simulink model "PowerWindowControl_V6"  (R2021a)
settings: Solver=VariableStepAuto  StartTime=0.0  StopTime=40  RelTol=1e-3
model workspace (MATLAB code in the model file):
  | testing=1;
undefined symbols (not defined in the file): sigbuilder_block
settings Model: VariantConfigurationObject=input_variant  EnablePacing=on  PacingRate=0.630000  Creator=achu  LastModifiedBy=achu

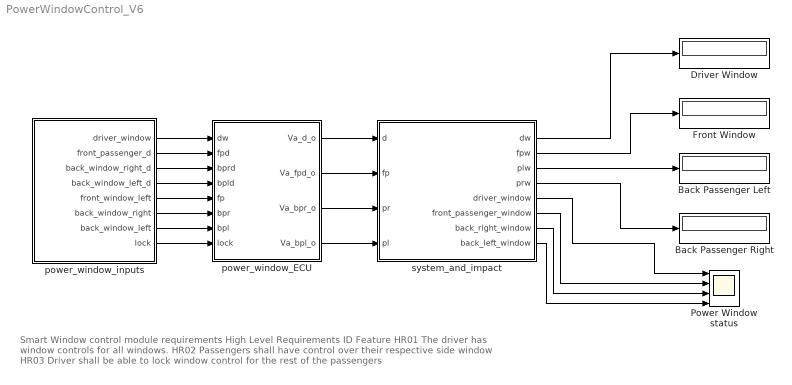
== system PowerWindowControl_V6 ==
  note: Smart Window control module requirements
      |
      | High Level Requirements
      |
      | ID
      | Feature
      |
      | HR01
      | The driver has window controls for all windows.
      |
      | HR02
      | Passengers shall have control over their respective side window
      |
      | HR03
      | Driver shall be able to lock window control for the rest of the passengers
  Back Passenger Left : Display
  Back Passenger Right : Display
  Driver Window : Display
  Front Window : Display
  Power Window status : Scope  NumInputPorts=4
  power_window_ECU : Subsystem
  power_window_inputs : Subsystem
  system_and_impact : Subsystem
  wires:
  system_and_impact/1(dw) -> Driver Window/1
  system_and_impact/4(prw) -> Back Passenger Right/1
  system_and_impact/2(fpw) -> Front Window/1
  system_and_impact/3(plw) -> Back Passenger Left/1
  system_and_impact/6(front_passenger_window) -> Power Window status/2
  system_and_impact/5(driver_window) -> Power Window status/1
  system_and_impact/7(back_right_window) -> Power Window status/3
  system_and_impact/8(back_left_window) -> Power Window status/4
  power_window_ECU/1(Va_d_o) -> system_and_impact/1(d)
  power_window_ECU/2(Va_fpd_o) -> system_and_impact/2(fp)
  power_window_ECU/3(Va_bpr_o) -> system_and_impact/3(pr)
  power_window_ECU/4(Va_bpl_o) -> system_and_impact/4(pl)
  power_window_inputs/1(driver_window) -> power_window_ECU/1(dw)
  power_window_inputs/2(front_passenger_d) -> power_window_ECU/2(fpd)
  power_window_inputs/3(back_window_right_d) -> power_window_ECU/3(bprd)
  power_window_inputs/4(back_window_left_d) -> power_window_ECU/4(bpld)
  power_window_inputs/5(front_window_left) -> power_window_ECU/5(fp)
  power_window_inputs/6(back_window_right) -> power_window_ECU/6(bpr)
  power_window_inputs/7(back_window_left) -> power_window_ECU/7(bpl)
  power_window_inputs/8(lock) -> power_window_ECU/8(lock)

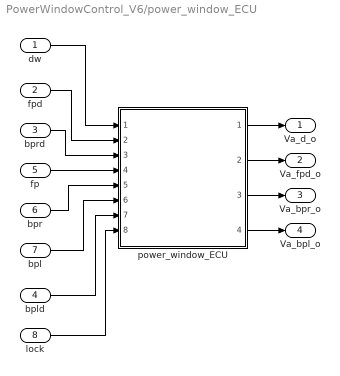
== system PowerWindowControl_V6/power_window_ECU ==
  dw : Inport
  fpd : Inport  Port=2
  bprd : Inport  Port=3
  bpld : Inport  Port=4
  fp : Inport  Port=5
  bpr : Inport  Port=6
  bpl : Inport  Port=7
  lock : Inport  Port=8
  power_window_ECU : Subsystem  ReferencedSubsystem=power_windows_ECU
  Va_d_o : Outport
  Va_fpd_o : Outport  Port=2
  Va_bpr_o : Outport  Port=3
  Va_bpl_o : Outport  Port=4
  wires:
  fp/1 -> power_window_ECU/4
  power_window_ECU/4 -> Va_bpl_o/1
  bprd/1 -> power_window_ECU/3
  dw/1 -> power_window_ECU/1
  bpr/1 -> power_window_ECU/5
  fpd/1 -> power_window_ECU/2
  power_window_ECU/2 -> Va_fpd_o/1
  lock/1 -> power_window_ECU/8
  bpl/1 -> power_window_ECU/6
  bpld/1 -> power_window_ECU/7
  power_window_ECU/3 -> Va_bpr_o/1
  power_window_ECU/1 -> Va_d_o/1

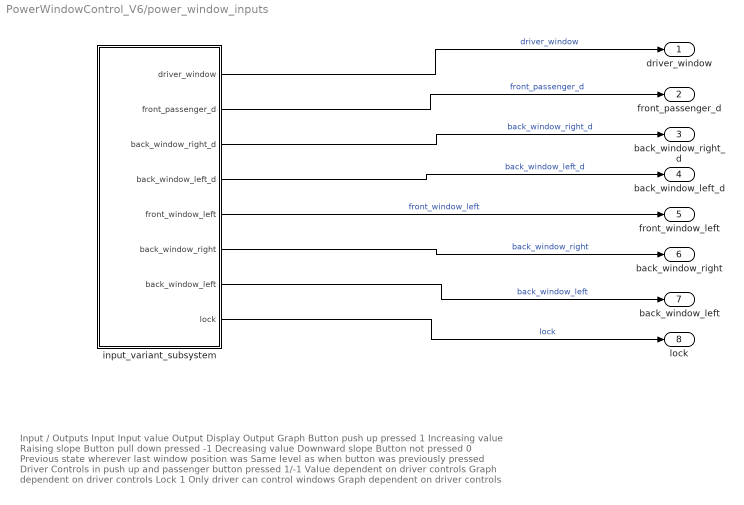
== system PowerWindowControl_V6/power_window_inputs ==
  note: Input / Outputs
      |
      | Input
      | Input value
      | Output Display
      | Output Graph
      |
      | Button push up pressed
      | 1
      | Increasing value
      | Raising slope
      |
      | Button pull down pressed
      | -1
      | Decreasing value
      | Downward slope
      |
      | Button not pressed
      | 0
      | Previous state wherever last window position was
      | Same level as when button was previously pressed
      |
      | Driver Controls in push up and passenger button pressed
      | 1/-1
      | Value dependent on driver controls
      | Graph dependent on driver controls
      |
      | Lock
      | 1
      | Only driver can control windows
      | Graph dependent on driver controls
  input_variant_subsystem : Subsystem  Variant=on
  driver_window : Outport
  front_passenger_d : Outport  Port=2
  back_window_right_d : Outport  Port=3
  back_window_left_d : Outport  Port=4
  front_window_left : Outport  Port=5
  back_window_right : Outport  Port=6
  back_window_left : Outport  Port=7
  lock : Outport  Port=8
  wires:
  input_variant_subsystem/4(back_window_left_d) -> back_window_left_d/1  "back_window_left_d"
  input_variant_subsystem/6(back_window_right) -> back_window_right/1  "back_window_right"
  input_variant_subsystem/7(back_window_left) -> back_window_left/1  "back_window_left"
  input_variant_subsystem/1(driver_window) -> driver_window/1  "driver_window"
  input_variant_subsystem/5(front_window_left) -> front_window_left/1  "front_window_left"
  input_variant_subsystem/3(back_window_right_d) -> back_window_right_d/1  "back_window_right_d"
  input_variant_subsystem/8(lock) -> lock/1  "lock"
  input_variant_subsystem/2(front_passenger_d) -> front_passenger_d/1  "front_passenger_d"

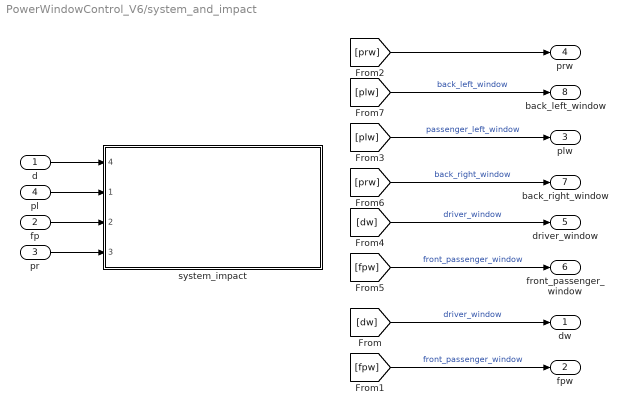
== system PowerWindowControl_V6/system_and_impact ==
  d : Inport
  fp : Inport  Port=2
  pr : Inport  Port=3
  pl : Inport  Port=4
  system_impact : Subsystem  ReferencedSubsystem=power_window_system_impact
      settings: PortSchema="{\"entries\":[{\"content\":{\"sides\":[{\"content\":{\"connectorIds\":[\"In4\",\"In1\",\"In2\",\"In3\"]},\"type\":\"ConnectorPlacement.EquallySpacedRectSide\",\"uuid\":\"b569c369-6bf1-43ff-8879-a618619a733c\"},{\"content\":{\"connectorIds\":[],\"side\":\"RIGHT\"},\"type\":\"ConnectorPlacement.EquallySpacedRectSide\",\"uuid\":\"d2d8ce62-aa5e-467c-813a-b2eb407d7f29\"},{\"content\":{\"connectorIds\":[],\"side\":\"TOP\"},\"type\":\"ConnectorPlacement.EquallySpacedRectSide\",\"uuid\":\"ba3f0d8f-c0c9-48ab-af13-329858e1637f\"}]},\"type\":\"ConnectorPlacement.EquallySpacedConnector\",\"uuid\":\"856bf121-72aa-430a-8fbb-3ccc8c554556\"}],\"packageUris\":[\"http://schema.mathworks.com/mf0/Connector/R2020b\"],\"version\":\"1.0\"}"
  dw : Outport
  fpw : Outport  Port=2
  plw : Outport  Port=3
  prw : Outport  Port=4
  driver_window : Outport  Port=5
  front_passenger_window : Outport  Port=6
  back_right_window : Outport  Port=7
  back_left_window : Outport  Port=8
  wires:
  [fpw] -> fpw/1  "front_passenger_window"
  [prw] -> back_right_window/1  "back_right_window"
  [plw] -> plw/1  "passenger_left_window"
  [dw] -> dw/1  "driver_window"
  [prw] -> prw/1
  [dw] -> driver_window/1  "driver_window"
  [plw] -> back_left_window/1  "back_left_window"
  [fpw] -> front_passenger_window/1  "front_passenger_window"
  pr/1 -> system_impact/3
  fp/1 -> system_impact/2
  pl/1 -> system_impact/1
  d/1 -> system_impact/4

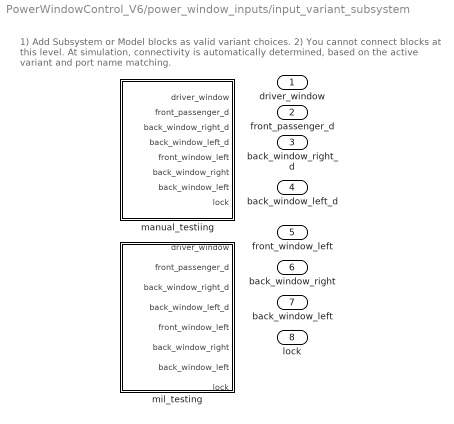
== system PowerWindowControl_V6/power_window_inputs/input_variant_subsystem ==
  note: 1) Add Subsystem or Model blocks as valid variant choices.
      | 2) You cannot connect blocks at this level. At simulation, connectivity is automatically
      | determined, based on the active variant and port name matching.
  manual_testiing : Subsystem  VariantControl=Choice
  mil_testing : Subsystem  VariantControl=Choice_1
  driver_window : Outport
  front_passenger_d : Outport  Port=2
  back_window_right_d : Outport  Port=3
  back_window_left_d : Outport  Port=4
  front_window_left : Outport  Port=5
  back_window_right : Outport  Port=6
  back_window_left : Outport  Port=7
  lock : Outport  Port=8

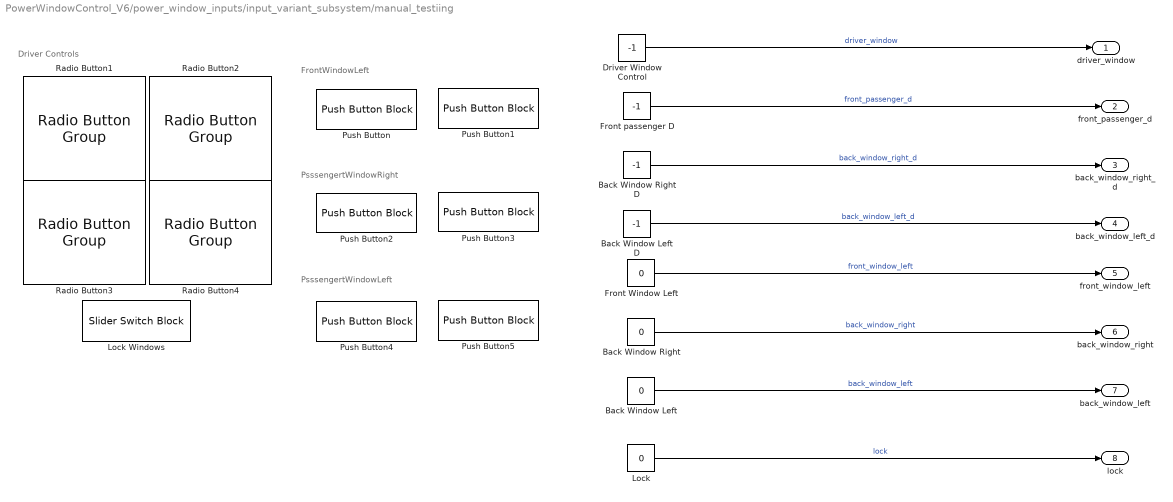
== system PowerWindowControl_V6/power_window_inputs/input_variant_subsystem/manual_testiing ==
  note: PsssengertWindowLeft
  note: PsssengertWindowRight
  note: Driver Controls
  note: FrontWindowLeft
  Back Window Left : Constant  Value=0
  Back Window Left D : Constant  Value=-1
  Back Window Right : Constant  Value=0
  Back Window Right D : Constant  Value=-1
  Driver Window Control : Constant  Value=-1
  Front Window Left : Constant  Value=0
  Front passenger D : Constant  Value=-1
  Lock : Constant  Value=0
  Lock Windows : SliderSwitchBlock
      settings: Values={{'Unlock', 'Lock'}, [0 1]}
  Push Button : PushButtonBlock  ButtonText=Push up window
  Push Button1 : PushButtonBlock  ButtonText=Pull down window  OnValue=-1
  Push Button2 : PushButtonBlock  ButtonText=Push up window
  Push Button3 : PushButtonBlock  ButtonText=Pull down window  OnValue=-1
  Push Button4 : PushButtonBlock  ButtonText=Push up window
  Push Button5 : PushButtonBlock  ButtonText=Pull down window  OnValue=-1
  Radio Button1 : RadioButtonGroup  LabelPosition=Hide  SelectedLabel=Close  ButtonGroupName=Driver Window Controls
      settings: Values={{'Open', 'Stop', 'Close'}, [1 0 -1]}
  Radio Button2 : RadioButtonGroup  LabelPosition=Hide  SelectedLabel=Close  ButtonGroupName=Front Passenger
      settings: Values={{'Open', 'Stop', 'Close'}, [1 0 -1]}
  Radio Button3 : RadioButtonGroup  LabelPosition=Hide  SelectedLabel=Close  ButtonGroupName=Back Window Right
      settings: Values={{'Open', 'Stop', 'Close'}, [1 0 -1]}
  Radio Button4 : RadioButtonGroup  LabelPosition=Hide  SelectedLabel=Close  ButtonGroupName=Back Window Left
      settings: Values={{'Open', 'Stop', 'Close'}, [1 0 -1]}
  driver_window : Outport
  front_passenger_d : Outport  Port=2
  back_window_right_d : Outport  Port=3
  back_window_left_d : Outport  Port=4
  front_window_left : Outport  Port=5
  back_window_right : Outport  Port=6
  back_window_left : Outport  Port=7
  lock : Outport  Port=8
  wires:
  Front passenger D/1 -> front_passenger_d/1  "front_passenger_d"
  Lock/1 -> lock/1  "lock"
  Front Window Left/1 -> front_window_left/1  "front_window_left"
  Driver Window Control/1 -> driver_window/1  "driver_window"
  Back Window Right D/1 -> back_window_right_d/1  "back_window_right_d"
  Back Window Left/1 -> back_window_left/1  "back_window_left"
  Back Window Right/1 -> back_window_right/1  "back_window_right"
  Back Window Left D/1 -> back_window_left_d/1  "back_window_left_d"

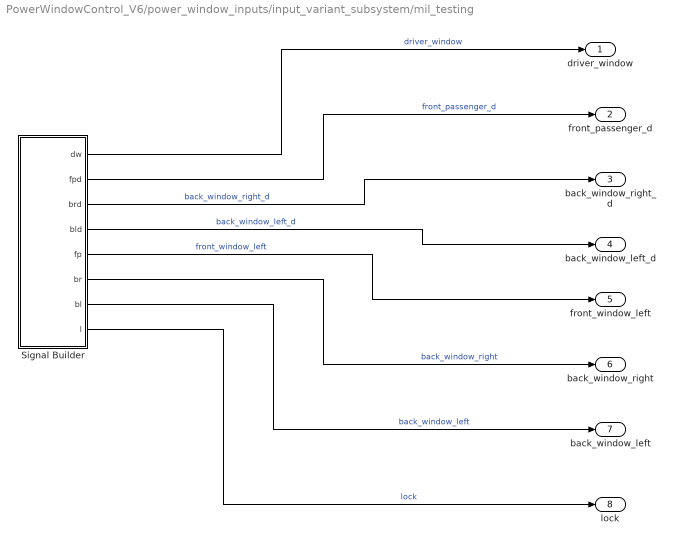
== system PowerWindowControl_V6/power_window_inputs/input_variant_subsystem/mil_testing ==
  Signal Builder : Subsystem  Tag=STV Subsys  LoadFcn=sigbuilder_block('load');  StartFcn=sigbuilder_block('start');  StopFcn=sigbuilder_block('stop');  ClipboardFcn=sigbuilder_block('clipboard');  mask(Sigbuilder block){tuvar=[0:10]}
      mask help: Simulink:masks:SigbuilderBlock_MD
      mask init:
      | if ~strcmp(get_param(bdroot(gcbh),'SimulationStatus'),'stopped') tuvar = sigbuilder_block('maskInit'); end
      settings: CopyFcn=sigbuilder_block('copy');  DeleteFcn=sigbuilder_block('delete');  ModelCloseFcn=sigbuilder_block('modelClose');  PreSaveFcn=sigbuilder_block('preSave');  PauseFcn=sigbuilder_block('pause');  ContinueFcn=sigbuilder_block('continue');  NameChangeFcn=sigbuilder_block('namechange');  OpenFcn=sigbuilder_block('open',[437.6 199.2 550.4 400 ]);  CloseFcn=sigbuilder_block('close');
      mask Display: plot(0, 0, 100, 100,[2, 2, 32, 32, 2], [68, 8, 8, 68, 68],[32, 2], [38, 38], [32, 19, 2],[53, 60, 44], [32, 17, 17, 2],[16, 16, 31, 31]);txt = getActiveGroup(gcbh);text(2, 100, txt,'verticalAlignment', 'top');
  driver_window : Outport
  front_passenger_d : Outport  Port=2
  back_window_right_d : Outport  Port=3
  back_window_left_d : Outport  Port=4
  front_window_left : Outport  Port=5
  back_window_right : Outport  Port=6
  back_window_left : Outport  Port=7
  lock : Outport  Port=8
  wires:
  Signal Builder/5(fp) -> front_window_left/1  "front_window_left"
  Signal Builder/7(bl) -> back_window_left/1  "back_window_left"
  Signal Builder/8(l) -> lock/1  "lock"
  Signal Builder/3(brd) -> back_window_right_d/1  "back_window_right_d"
  Signal Builder/6(br) -> back_window_right/1  "back_window_right"
  Signal Builder/1(dw) -> driver_window/1  "driver_window"
  Signal Builder/2(fpd) -> front_passenger_d/1  "front_passenger_d"
  Signal Builder/4(bld) -> back_window_left_d/1  "back_window_left_d"

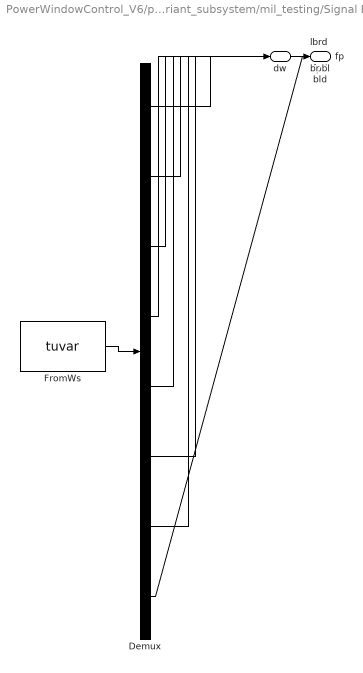
== system PowerWindowControl_V6/power_window_inputs/input_variant_subsystem/mil_testing/Signal Builder ==
  Demux : Demux  Tag=STV Demux  Outputs=8
      settings: DisplayOption=none
  FromWs : FromWorkspace  Tag=STV FromWs  VariableName=tuvar
      SigBuilderData=|
      | common.afterFinalStr = 'Extrapolate'
      | common.sampleTime = 0
      | dataSet.timeRange = [0 20]
      | dataSet.name = 'Sheet1'
      | sbobj.Name = 'Signal Builder'
      | sbobj.Groups.Name = 'Sheet1'
      | sbobj.Groups.Signals(1).Name = 'dw'
      | sbobj.Groups.Signals(1).XData = [0 1 2 3 4 5 6 7 8 9 10 11 12 13 14 15 16 17 18 19 20]
      | sbobj.Groups.Signals(1).YData = [0 1 1 1 0 0 0 0 -1 -1 -1 -1 -1 1 1 1 1 0 0 0 0]
      | sbobj.Groups.Signals(2).Name = 'fpd'
      | sbobj.Groups.Signals(2).XData = [0 1 2 3 4 5 6 7 8 9 10 11 12 13 14 15 16 17 18 19 20]
      | sbobj.Groups.Signals(2).YData = [0 1 1 -1 -1 -1 1 1 1 1 1 0 0 0 0 0 0 0 0 0 0]
      | sbobj.Groups.Signals(3).Name = 'brd'
      | sbobj.Groups.Signals(3).XData = [0 1 2 3 4 5 6 7 8 9 10 11 12 13 14 15 16 17 18 19 20]
      | sbobj.Groups.Signals(3).YData = [0 1 1 1 1 -1 -1 -1 -1 -1 -1 0 0 0 0 0 0 0 0 0 0]
      | sbobj.Groups.Signals(4).Name = 'bld'
      | sbobj.Groups.Signals(4).XData = [0 1 2 3 4 5 6 7 8 9 10 11 12 13 14 15 16 17 18 19 20]
      | sbobj.Groups.Signals(4).YData = [0 1 1 1 1 -1 -1 -1 -1 -1 1 1 1 0 0 0 0 0 0 0 0]
      | sbobj.Groups.Signals(5).Name = 'fp'
      | sbobj.Groups.Signals(5).XData = [0 1 2 3 4 5 6 7 8 9 10 11 12 13 14 15 16 17 18 19 20]
      | sbobj.Groups.Signals(5).YData = [0 -1 -1 1 1 1 -1 -1 -1 -1 -1 -1 -1 -1 1 1 1 1 1 1 1]
      | sbobj.Groups.Signals(6).Name = 'br'
      | sbobj.Groups.Signals(6).XData = [0 1 2 3 4 5 6 7 8 9 10 11 12 13 14 15 16 17 18 19 20]
      | sbobj.Groups.Signals(6).YData = [0 -1 -1 -1 -1 1 1 -1 -1 1 1 1 1 -1 -1 -1 -1 1 1 1 1]
      | sbobj.Groups.Signals(7).Name = 'bl'
      | sbobj.Groups.Signals(7).XData = [0 1 2 3 4 5 6 7 8 9 10 11 12 13 14 15 16 17 18 19 20]
      | sbobj.Groups.Signals(7).YData = [0 1 1 0 0 1 1 0 0 1 1 -1 -1 -1 -1 -1 -1 1 1 1 1]
      | sbobj.Groups.Signals(8).Name = 'l'
      | sbobj.Groups.Signals(8).XData = [0 1 2 3 4 5 6 7 8 9 10 11 12 13 14 15 16 17 18 19 20]
      | sbobj.Groups.Signals(8).YData = [0 0 0 0 0 0 1 1 1 1 1 1 1 1 0 0 0 0 0 0 0]
      | sbobj.Groups.TimeRange = [0 20]
  dw : Outport  Tag=STV Outport
  fpd : Outport  Tag=STV Outport  Port=2
  brd : Outport  Tag=STV Outport  Port=3
  bld : Outport  Tag=STV Outport  Port=4
  fp : Outport  Tag=STV Outport  Port=5
  br : Outport  Tag=STV Outport  Port=6
  bl : Outport  Tag=STV Outport  Port=7
  l : Outport  Tag=STV Outport  Port=8
  wires:
  Demux/1 -> dw/1
  FromWs/1 -> Demux/1
  Demux/2 -> fpd/1
  Demux/3 -> brd/1
  Demux/4 -> bld/1
  Demux/5 -> fp/1
  Demux/6 -> br/1
  Demux/7 -> bl/1
  Demux/8 -> l/1
